simulink model "simulink_non"  (R2020b)
settings: Solver=VariableStepAuto  StartTime=0.0  StopTime=40  RelTol=1e-3
values from neighbouring files (symbols this model uses):
  A = double(Fp(0,0,0,0))    [Main.m]
  B = double(jacobian(F,u))    [Main.m]
  C = [1 0 0 0]    [Main.m]
  D = 0    [Main.m]
settings Model: Creator=Javad  LastModifiedBy=Javad

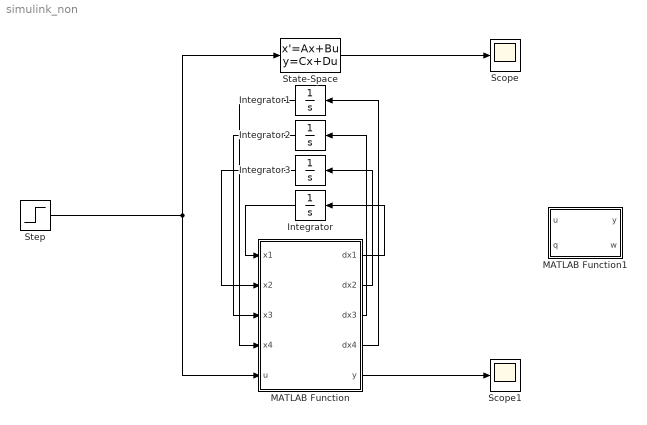
== system simulink_non ==
  Integrator{,1..3} (4 alike) : Integrator
  MATLAB Function : MATLAB Function  TreatAsAtomicUnit=on
  MATLAB Function1 : MATLAB Function  TreatAsAtomicUnit=on
  Scope : Scope
  Scope1 : Scope
  State-Space : StateSpace  A=A  B=B  C=C  D=D  InitialCondition=0
  Step : Step  SampleTime=0
  wires:
  State-Space/1 -> Scope/1
  Step/1 -> State-Space/1, MATLAB Function/5(u)
  MATLAB Function/1(dx1) -> Integrator/1
  Integrator/1 -> MATLAB Function/1(x1)
  MATLAB Function/2(dx2) -> Integrator3/1
  Integrator3/1 -> MATLAB Function/2(x2)
  MATLAB Function/3(dx3) -> Integrator2/1
  Integrator2/1 -> MATLAB Function/3(x3)
  Integrator1/1 -> MATLAB Function/4(x4)
  MATLAB Function/4(dx4) -> Integrator1/1
  MATLAB Function/5(y) -> Scope1/1

== matlab function simulink_non/MATLAB Function1 ==
  data: u input; y output; q input; w output
function [y,w] = fcn(u,q)

y = u;

== matlab function simulink_non/MATLAB Function ==
  data: dx1 output; dx2 output; dx3 output; dx4 output; x1 input; x2 input; x3 input; x4 input; u input; y output
function [dx1,dx2,dx3,dx4,y] = fcn(x1,x2,x3,x4,u)
dx1=x2;
dx2=x3;
dx3=x4;
dx4=-2.344*x1-15.03*x2-26.19*x3-14.50*x4+x1*x3+x4^2+x2^2*(1+x2^2)^(1/2)+u;
y = x1;
